simulink model "my_twohoists"  (Simulink 9.2)
settings: Solver=FixedStepDiscrete  StartTime=0.0  StopTime=5400  FixedStep=sampleTime  RelTol=1e-3  EnableMultiTasking=on
libraries: vrlib x1
settings Model: Creator=jules  LastModifiedBy=jules
settings OptimizationCC: InitFltsAndDblsToZero=on
settings DebuggingCC: SaveWithParameterizedLinksMsg=none  SignalResolutionControl=TryResolveAllWithWarning  SolverPrmCheckMsg=warning  MultiTaskDSMMsg=warning  MultiTaskCondExecSysMsg=none  StateNameClashWarn=none
settings SFSimCC: SimUseLocalCustomCode=on
settings RTWCC: RTWUseLocalCustomCode=on
settings GRTTargetCC: TargetFcnLib=ansi_tfl_tmw.mat  GeneratePreprocessorConditionals=Use local settings
settings ConfigComp: CovExternalEMLEnable=on

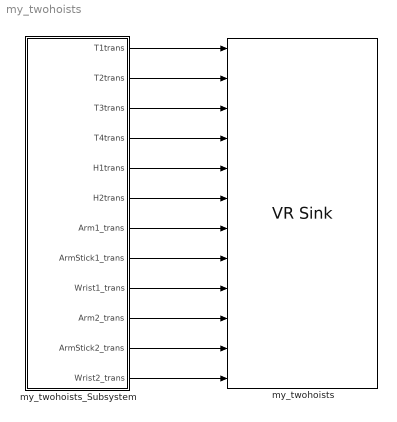
== system my_twohoists ==
  my_twohoists : vrlib/VR Sink  InstantiateOnLoad=on  SampleTime=1  ViewEnable=on  RemoteChange=off  RemoteView=on  FieldsWritten=T1.translation.3.1.double#T2.translation.3.1.double#T3.translation.3.1.double#T4.translation.3.1.double#Hoist1.translation.3.1.double#Hoist2.translation.3.1.double#Arm1.translation.3.1.double#ArmStick1.height.1.1.double#Wrist1.translation.3.1.double#Arm2.translation.3.1.double#ArmStick2.height.1.1.double#Wrist2.translation.3.1.double#  WorldFileName=my_twohoists.wrl  AutoView=on  VideoDimensions=[]  AllowVariableSize=off  FigureProperties="{'Position', 'Name', 'Viewpoint', 'CameraBound', 'CameraDirection', 'CameraPosition', 'CameraUpVector', 'ZoomFactor', 'Antialiasing', 'Headlight', 'Lighting', 'NavPanel', 'Sound', 'StatusBar', 'Stereo3D', 'Stereo3DCameraOffset', 'Stereo3DHIT', 'ToolBar', 'Textures', 'Transparency', 'Triad', 'Wireframe', 'NavZones', 'NavMode', 'NavSpeed', 'CaptureFileFormat', 'CaptureFileName', 'Record2DCompressMethod', 'Record2DCompressQuality', 'Record2D', 'Record2DFileName', 'Record2DFPS'; [5.0000000000000000e+00   7.5000000000000000e+01   1.2700000000000000e+03   3.5000000000000000e+02], 'Hoist', 'View1', 'on', [0.0000000000000000e+00   0.0000000000000000e+00  -1.0000000000000000e+00], [0.0000000000000000e+00   0.0000000000000000e+00   0.0000000000000000e+00], [0.0000000000000000e+00   1.0000000000000000e+00   0.0000000000000000e+00], [1.0000000000000000e+00], 'on', 'on', 'on', 'halfbar', 'on', 'on', 'off', [1.0000000149011612e-01], [0.0000000000000000e+00], 'on', 'on', 'on', 'none', 'off', 'off', 'fly', 'normal', 'tif', '%f_anim_%n.tif', 'auto', [7.5000000000000000e+01], 'off', '%f_anim_%n.avi', 'auto'}"
      settings: SourceProductBaseCode=VR
  my_twohoists_Subsystem : Subsystem
  wires:
  my_twohoists_Subsystem/1(T1trans) -> my_twohoists/1
  my_twohoists_Subsystem/2(T2trans) -> my_twohoists/2
  my_twohoists_Subsystem/3(T3trans) -> my_twohoists/3
  my_twohoists_Subsystem/4(T4trans) -> my_twohoists/4
  my_twohoists_Subsystem/5(H1trans) -> my_twohoists/5
  my_twohoists_Subsystem/6(H2trans) -> my_twohoists/6
  my_twohoists_Subsystem/7(Arm1_trans) -> my_twohoists/7
  my_twohoists_Subsystem/8(ArmStick1_trans) -> my_twohoists/8
  my_twohoists_Subsystem/9(Wrist1_trans) -> my_twohoists/9
  my_twohoists_Subsystem/10(Arm2_trans) -> my_twohoists/10
  my_twohoists_Subsystem/11(ArmStick2_trans) -> my_twohoists/11
  my_twohoists_Subsystem/12(Wrist2_trans) -> my_twohoists/12

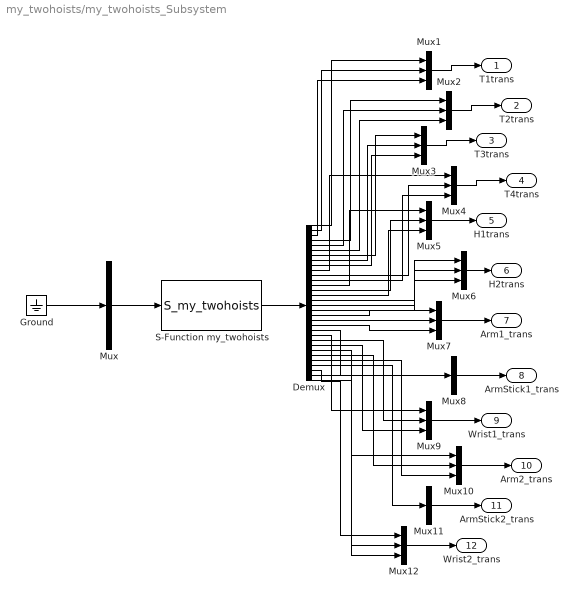
== system my_twohoists/my_twohoists_Subsystem ==
  Demux : Demux  Outputs=32
  Ground : Ground
  Mux : Mux  Inputs=1
  Mux{1..7,9..10,12} (10 alike) : Mux  Inputs=3
  Mux11 : Mux  Inputs=1
  Mux8 : Mux  Inputs=1
  S-Function my_twohoists : S-Function  FunctionName=S_my_twohoists  Parameters='my_twohoists.wrl',sampleTime,T,period  SFunctionDeploymentMode=off  EnableBusSupport=off
  T1trans : Outport
  T2trans : Outport  Port=2
  T3trans : Outport  Port=3
  T4trans : Outport  Port=4
  H1trans : Outport  Port=5
  H2trans : Outport  Port=6
  Arm1_trans : Outport  Port=7
  ArmStick1_trans : Outport  Port=8
  Wrist1_trans : Outport  Port=9
  Arm2_trans : Outport  Port=10
  ArmStick2_trans : Outport  Port=11
  Wrist2_trans : Outport  Port=12
  wires:
  Mux/1 -> S-Function my_twohoists/1
  S-Function my_twohoists/1 -> Demux/1
  Ground/1 -> Mux/1
  Mux1/1 -> T1trans/1
  Demux/1 -> Mux1/1
  Demux/2 -> Mux1/2
  Demux/3 -> Mux1/3
  Mux2/1 -> T2trans/1
  Mux3/1 -> T3trans/1
  Mux4/1 -> T4trans/1
  Mux5/1 -> H1trans/1
  Demux/4 -> Mux2/1
  Demux/5 -> Mux2/2
  Demux/7 -> Mux3/1
  Demux/8 -> Mux3/2
  Demux/9 -> Mux3/3
  Demux/10 -> Mux4/1
  Demux/11 -> Mux4/2
  Demux/12 -> Mux4/3
  Demux/13 -> Mux5/1
  Demux/14 -> Mux5/2
  Demux/15 -> Mux5/3
  Mux6/1 -> H2trans/1
  Demux/16 -> Mux6/1
  Demux/17 -> Mux6/2
  Demux/18 -> Mux6/3
  Mux7/1 -> Arm1_trans/1
  Demux/19 -> Mux7/1
  Demux/20 -> Mux7/2
  Demux/21 -> Mux7/3
  Mux8/1 -> ArmStick1_trans/1
  Mux9/1 -> Wrist1_trans/1
  Demux/22 -> Mux8/1
  Mux10/1 -> Arm2_trans/1
  Mux11/1 -> ArmStick2_trans/1
  Mux12/1 -> Wrist2_trans/1
  Demux/6 -> Mux2/3
  Demux/23 -> Mux9/1
  Demux/24 -> Mux9/2
  Demux/25 -> Mux9/3
  Demux/26 -> Mux10/1
  Demux/27 -> Mux10/2
  Demux/28 -> Mux10/3
  Demux/29 -> Mux11/1
  Demux/30 -> Mux12/1
  Demux/31 -> Mux12/2
  Demux/32 -> Mux12/3
